simulink model "d_014"  (Simulink 5.1)
settings: Solver=ode45  StartTime=0.0  StopTime=10.0  RelTol=1e-3
libraries: fm_lib x30
settings Model: Creator=fmilano  LastModifiedBy=fmilano  ExtModeAutoUpdateStatusClock=off  SignalLoggingName=logsout  RTWOptions="-aEnforceIntegerDowncast=1 -aFoldNonRolledExpr=1 -aInlineInvariantSignals=1 -aInlineParameters=0 -aLocalBlockOutputs=1 -aRollThreshold=5 -aZeroInternalMemoryAtStartup=1 -aZeroExternalMemoryAtStartup=1 -aInitFltsAndDblsToZero=1 -aForceBlockIOInitOptimize=0 -aGenerateReport=0 -aGenCodeOnly=0 -aRTWVerbose=1 -aIncludeHyperlinkInReport=0 -aLaunchReport=0 -aGenerateTraceInfo=0  -aForceParamTrailComments=0 -aGenerateComments=1 -aIgnoreCustomStorageClasses=1 -aIncHierarchyInIds=0 -aMaxRTWIdLen=31 -aShowEliminatedStatements=0 -aIncDataTypeInIds=0 -aInsertBlockDesc=0 -aIgnoreTestpoints=0 -aSimulinkBlockComments=1 -aInlinedPrmAccess=\"Literals\"  -aSuppressErrorStatus=0 -aModelReferenceCompliant=1 -aParenthesesLevel=\"Nominal\" -aModelStepFunctionPrototypeControlCompliant=0 -aPortableWordSizes=0 -aParMdlRefBuildCompliant=0 -aSupportNonInlinedSFcns=1 -aSupportContinuousTime=1 -aSupportComplex=1 -aSupportNonFinite=1 -aSupportAbsoluteTime=1 -aMultiwordLength=2048 -aTargetPreCompLibLocation=\"\" -aTargetLibSuffix=\"\" -aTargetFunctionLibrary=\"ANSI_C\" -aTargetFcnLib=\"ansi_tfl_tmw.mat\" -aMultiInstanceERTCode=0 -aLogVarNameModifier=\"rt_\" -aERTFirstTimeCompliant=0 -aIsPILTarget=0 -aCombineOutputUpdateFcns=0 -aGenerateASAP2=0 -aGenerateClassInterface=0 -aGenerateTestInterfaces=0 -aGenerateSampleERTMain=0 -aGenerateFullHeader=1 -aUtilityFuncGeneration=\"Auto\" -aIncludeFileDelimiter=\"Auto\" -aIncludeMdlTerminateFcn=1 -aPurelyIntegerCode=0 -aAutosarCompliant=0 -aERTCustomFileBanners=0 -aRTWCAPIStates=0 -aRTWCAPIParams=0 -aRTWCAPISignals=0 -aMatFileLogging=1 -aCompOptLevelCompliant=0 -aCPPClassGenCompliant=0 -aExtModeIntrfLevel=\"Level1\" -aExtModeMexFile=\"ext_comm\" -aExtModeTransport=0 -aExtModeStaticAllocSize=1000000 -aExtModeTesting=0 -aExtModeStaticAlloc=0 -aExtMode=0 -aERTMultiwordLength=256 -aERTMultiwordTypeDef=\"System defined\"  -aGenerateTraceInfo=0 -aGenerateTraceInfo=0 -aGenerateTraceInfo=0 -aGenerateTraceInfo=0 -aPrefixModelToSubsysFcnNames=1 -aGenerateASAP2=0 -aRTWCAPIStates=0 -aRTWCAPIParams=0 -aRTWCAPISignals=0 -aExtModeMexFile=\"ext_comm\" -aExtModeTransport=0 -aExtModeStaticAllocSize=1000000 -aExtModeTesting=0 -aExtModeStaticAlloc=0 -aExtMode=0"

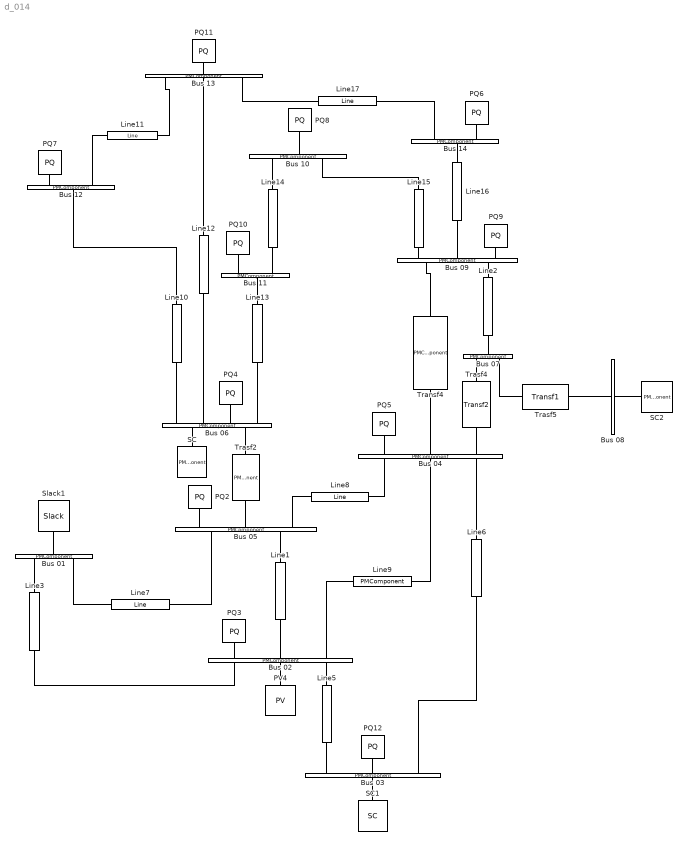
== system d_014 ==
  Bus 01 : PMComponent  Tag=PSATblock  Description=Connection  Orientation=down  PhysicalDomain=psatdomain  LeftPortType=p1  RightPortType=p1  LConnTagsString=__newl0  RConnTagsString=__newr0|__newr1  mask(Bus){in=1, out=2, p2q=69, p3_4q=[1.00  0.00], p5q=4, p6q=1}
      mask prompts: in "Number of inputs:"; out "Number of outputs:"; p2q "Voltage Rating [kV]"; p3_4q "Voltage initial guess [p.u.  rad]"; p5q "Area number"; p6q "Region number"
      mask help: Bus block.
      mask init:
      | fm_inout
      mask CallbackString: ||||fm_block|
      mask Display: plot([0 1 1 0 0],[0 0 1 1 0])
  Bus 02 : PMComponent  Tag=PSATblock  Description=Connection  Orientation=up  PhysicalDomain=psatdomain  LeftPortType=p1  RightPortType=p1  LConnTagsString=__newl0|__newl1|__newl2  RConnTagsString=__newr0|__newr1|__newr2  mask(Bus){in=3, out=3, p2q=69, p3_4q=[1.00  0.00], p5q=4, p6q=1}
      mask prompts: in "Number of inputs:"; out "Number of outputs:"; p2q "Voltage Rating [kV]"; p3_4q "Voltage initial guess [p.u.  rad]"; p5q "Area number"; p6q "Region number"
      mask help: Bus block.
      mask init:
      | fm_inout
      mask CallbackString: ||||fm_block|
      mask Display: plot([0 1 1 0 0],[0 0 1 1 0])
  Bus 03 : PMComponent  Tag=PSATblock  Description=Connection  Orientation=up  PhysicalDomain=psatdomain  LeftPortType=p1  RightPortType=p1  LConnTagsString=__newl0  RConnTagsString=__newr0|__newr1|__newr2  mask(Bus){in=1, out=3, p2q=69, p3_4q=[1.00  0.00], p5q=4, p6q=1}
      mask prompts: in "Number of inputs:"; out "Number of outputs:"; p2q "Voltage Rating [kV]"; p3_4q "Voltage initial guess [p.u.  rad]"; p5q "Area number"; p6q "Region number"
      mask help: Bus block.
      mask init:
      | fm_inout
      mask CallbackString: ||||fm_block|
      mask Display: plot([0 1 1 0 0],[0 0 1 1 0])
  Bus 04 : PMComponent  Tag=PSATblock  Description=Connection  Orientation=up  PhysicalDomain=psatdomain  LeftPortType=p1  RightPortType=p1  LConnTagsString=__newl0|__newl1|__newl2  RConnTagsString=__newr0|__newr1|__newr2  mask(Bus){in=3, out=3, p2q=69, p3_4q=[1.00  0.00], p5q=4, p6q=1}
      mask prompts: in "Number of inputs:"; out "Number of outputs:"; p2q "Voltage Rating [kV]"; p3_4q "Voltage initial guess [p.u.  rad]"; p5q "Area number"; p6q "Region number"
      mask help: Bus block.
      mask init:
      | fm_inout
      mask CallbackString: ||||fm_block|
      mask Display: plot([0 1 1 0 0],[0 0 1 1 0])
  Bus 05 : PMComponent  Tag=PSATblock  Description=Connection  Orientation=up  PhysicalDomain=psatdomain  LeftPortType=p1  RightPortType=p1  LConnTagsString=__newl0|__newl1  RConnTagsString=__newr0|__newr1|__newr2  mask(Bus){in=2, out=3, p2q=69, p3_4q=[1.00  0.00], p5q=4, p6q=1}
      mask prompts: in "Number of inputs:"; out "Number of outputs:"; p2q "Voltage Rating [kV]"; p3_4q "Voltage initial guess [p.u.  rad]"; p5q "Area number"; p6q "Region number"
      mask help: Bus block.
      mask init:
      | fm_inout
      mask CallbackString: ||||fm_block|
      mask Display: plot([0 1 1 0 0],[0 0 1 1 0])
  Bus 06 : PMComponent  Tag=PSATblock  Description=Connection  Orientation=up  PhysicalDomain=psatdomain  LeftPortType=p1  RightPortType=p1  LConnTagsString=__newl0|__newl1  RConnTagsString=__newr0|__newr1|__newr2|__newr3  mask(Bus){in=2, out=4, p2q=13.8, p3_4q=[1.00  0.00], p5q=2, p6q=1}
      mask prompts: in "Number of inputs:"; out "Number of outputs:"; p2q "Voltage Rating [kV]"; p3_4q "Voltage initial guess [p.u.  rad]"; p5q "Area number"; p6q "Region number"
      mask help: Bus block.
      mask init:
      | fm_inout
      mask CallbackString: ||||fm_block|
      mask Display: plot([0 1 1 0 0],[0 0 1 1 0])
  Bus 07 : PMComponent  Tag=PSATblock  Description=Connection  Orientation=up  PhysicalDomain=psatdomain  LeftPortType=p1  RightPortType=p1  LConnTagsString=__newl0|__newl1  RConnTagsString=__newr0  mask(Bus){in=2, out=1, p2q=13.8, p3_4q=[1.00  0.00], p5q=2, p6q=1}
      mask prompts: in "Number of inputs:"; out "Number of outputs:"; p2q "Voltage Rating [kV]"; p3_4q "Voltage initial guess [p.u.  rad]"; p5q "Area number"; p6q "Region number"
      mask help: Bus block.
      mask init:
      | fm_inout
      mask CallbackString: ||||fm_block|
      mask Display: plot([0 1 1 0 0],[0 0 1 1 0])
  Bus 08 : PMComponent  Tag=PSATblock  Description=Connection  Orientation=left  PhysicalDomain=psatdomain  LeftPortType=p1  RightPortType=p1  LConnTagsString=__newl0  RConnTagsString=__newr0  mask(Bus){in=1, out=1, p2q=18, p3_4q=[1.00  0.00], p5q=3, p6q=1}
      mask prompts: in "Number of inputs:"; out "Number of outputs:"; p2q "Voltage Rating [kV]"; p3_4q "Voltage initial guess [p.u.  rad]"; p5q "Area number"; p6q "Region number"
      mask help: Bus block.
      mask init:
      | fm_inout
      mask CallbackString: ||||fm_block|
      mask Display: plot([0 1 1 0 0],[0 0 1 1 0])
  Bus 09 : PMComponent  Tag=PSATblock  Description=Connection  Orientation=up  PhysicalDomain=psatdomain  LeftPortType=p1  RightPortType=p1  LConnTagsString=__newl0|__newl1  RConnTagsString=__newr0|__newr1|__newr2  mask(Bus){in=2, out=3, p2q=13.8, p3_4q=[1.00  0.00], p5q=2, p6q=1}
      mask prompts: in "Number of inputs:"; out "Number of outputs:"; p2q "Voltage Rating [kV]"; p3_4q "Voltage initial guess [p.u.  rad]"; p5q "Area number"; p6q "Region number"
      mask help: Bus block.
      mask init:
      | fm_inout
      mask CallbackString: ||||fm_block|
      mask Display: plot([0 1 1 0 0],[0 0 1 1 0])
  Bus 10 : PMComponent  Tag=PSATblock  Description=Connection  Orientation=up  PhysicalDomain=psatdomain  LeftPortType=p1  RightPortType=p1  LConnTagsString=__newl0|__newl1  RConnTagsString=__newr0  mask(Bus){in=2, out=1, p2q=13.8, p3_4q=[1.00  0.00], p5q=2, p6q=1}
      mask prompts: in "Number of inputs:"; out "Number of outputs:"; p2q "Voltage Rating [kV]"; p3_4q "Voltage initial guess [p.u.  rad]"; p5q "Area number"; p6q "Region number"
      mask help: Bus block.
      mask init:
      | fm_inout
      mask CallbackString: ||||fm_block|
      mask Display: plot([0 1 1 0 0],[0 0 1 1 0])
  Bus 11 : PMComponent  Tag=PSATblock  Description=Connection  Orientation=up  PhysicalDomain=psatdomain  LeftPortType=p1  RightPortType=p1  LConnTagsString=__newl0  RConnTagsString=__newr0|__newr1  mask(Bus){in=1, out=2, p2q=13.8, p3_4q=[1.00  0.00], p5q=2, p6q=1}
      mask prompts: in "Number of inputs:"; out "Number of outputs:"; p2q "Voltage Rating [kV]"; p3_4q "Voltage initial guess [p.u.  rad]"; p5q "Area number"; p6q "Region number"
      mask help: Bus block.
      mask init:
      | fm_inout
      mask CallbackString: ||||fm_block|
      mask Display: plot([0 1 1 0 0],[0 0 1 1 0])
  Bus 12 : PMComponent  Tag=PSATblock  Description=Connection  Orientation=up  PhysicalDomain=psatdomain  LeftPortType=p1  RightPortType=p1  LConnTagsString=__newl0  RConnTagsString=__newr0|__newr1  mask(Bus){in=1, out=2, p2q=13.8, p3_4q=[1.00  0.00], p5q=2, p6q=1}
      mask prompts: in "Number of inputs:"; out "Number of outputs:"; p2q "Voltage Rating [kV]"; p3_4q "Voltage initial guess [p.u.  rad]"; p5q "Area number"; p6q "Region number"
      mask help: Bus block.
      mask init:
      | fm_inout
      mask CallbackString: ||||fm_block|
      mask Display: plot([0 1 1 0 0],[0 0 1 1 0])
  Bus 13 : PMComponent  Tag=PSATblock  Description=Connection  Orientation=up  PhysicalDomain=psatdomain  LeftPortType=p1  RightPortType=p1  LConnTagsString=__newl0|__newl1|__newl2  RConnTagsString=__newr0  mask(Bus){in=3, out=1, p2q=13.8, p3_4q=[1.00  0.00], p5q=2, p6q=1}
      mask prompts: in "Number of inputs:"; out "Number of outputs:"; p2q "Voltage Rating [kV]"; p3_4q "Voltage initial guess [p.u.  rad]"; p5q "Area number"; p6q "Region number"
      mask help: Bus block.
      mask init:
      | fm_inout
      mask CallbackString: ||||fm_block|
      mask Display: plot([0 1 1 0 0],[0 0 1 1 0])
  Bus 14 : PMComponent  Tag=PSATblock  Description=Connection  Orientation=up  PhysicalDomain=psatdomain  LeftPortType=p1  RightPortType=p1  LConnTagsString=__newl0  RConnTagsString=__newr0|__newr1  mask(Bus){in=1, out=2, p2q=13.8, p3_4q=[1.00  0.00], p5q=2, p6q=1}
      mask prompts: in "Number of inputs:"; out "Number of outputs:"; p2q "Voltage Rating [kV]"; p3_4q "Voltage initial guess [p.u.  rad]"; p5q "Area number"; p6q "Region number"
      mask help: Bus block.
      mask init:
      | fm_inout
      mask CallbackString: ||||fm_block|
      mask Display: plot([0 1 1 0 0],[0 0 1 1 0])
  Line1 : fm_lib/Power Flow/Line  Tag=PSATblock  Description=Power Flow  Orientation=up  PhysicalDomain=psatdomain  SubClassName=unknown  LeftPortType=p1  RightPortType=p1  LConnTagsString=__newl0  RConnTagsString=__newr0  p3_4_5q="[100  69  60]"  p6q=0  p8q=0.05695  p9q=0.17388  p10q=0.034  p13_14_15q="[0.0  0.0  0.0]"  p16q=on
  Line10 : PMComponent  Tag=PSATblock  Description=Power Flow  Orientation=up  PhysicalDomain=psatdomain  LeftPortType=p1  RightPortType=p1  LConnTagsString=__newl0  RConnTagsString=__newr0  mask(Line){p3_4_5q=[100  13.8  60], p6q=0, p8q=0.12291, p9q=0.25581, p10q=0.00, p13_14_15q=[0.0  0.0  0.0], p16q=on}
      mask prompts: p3_4_5q "Power, Voltage and Frequency Ratings [MVA, kV, Hz]"; p6q "Length of line [km] (0 for p.u. parameters)"; p8q "Resistance [p.u. (Ohms/km)]"; p9q "Reactance [p.u. (H/km)]"; p10q "Susceptance [p.u. (F/km)]"; p13_14_15q "Imax, Pmax and Smax [p.u., p.u., p.u.]"; p16q "Connected"
      mask help: This block defines a pi model for a tree phase line.
      mask init:
      | [xp,yp] = fm_draw('pi');
      mask CallbackString: ||||||fm_block
      mask Display:
      | plot([-1  1  1 -1 -1],[-0.2 -0.2 0.2 0.2 -0.2])
      | color('blue')
      | plot(0.35*xp,0.2*yp)
  Line11 : fm_lib/Power Flow/Line  Tag=PSATblock  Description=Power Flow  PhysicalDomain=psatdomain  SubClassName=unknown  LeftPortType=p1  RightPortType=p1  LConnTagsString=__newl0  RConnTagsString=__newr0  p3_4_5q="[100  13.8  60]"  p6q=0  p8q=0.22092  p9q=0.19988  p10q=0.00  p13_14_15q="[0.0  0.0  0.0]"  p16q=on
  Line12 : fm_lib/Power Flow/Line  Tag=PSATblock  Description=Power Flow  Orientation=up  PhysicalDomain=psatdomain  SubClassName=unknown  LeftPortType=p1  RightPortType=p1  LConnTagsString=__newl0  RConnTagsString=__newr0  p3_4_5q="[100  13.8  60]"  p6q=0  p8q=0.06615  p9q=0.13027  p10q=0.00  p13_14_15q="[0.0  0.0  0.0]"  p16q=on
  Line13 : fm_lib/Power Flow/Line  Tag=PSATblock  Description=Power Flow  Orientation=up  PhysicalDomain=psatdomain  SubClassName=unknown  LeftPortType=p1  RightPortType=p1  LConnTagsString=__newl0  RConnTagsString=__newr0  p3_4_5q="[100  13.8  60]"  p6q=0  p8q=0.09498  p9q=0.1989  p10q=0.00  p13_14_15q="[0.0  0.0  0.0]"  p16q=on
  Line14 : fm_lib/Power Flow/Line  Tag=PSATblock  Description=Power Flow  Orientation=up  PhysicalDomain=psatdomain  SubClassName=unknown  LeftPortType=p1  RightPortType=p1  LConnTagsString=__newl0  RConnTagsString=__newr0  p3_4_5q="[100  13.8  60]"  p6q=0  p8q=0.08205  p9q=0.19207  p10q=0.00  p13_14_15q="[0.0  0.0  0.0]"  p16q=on
  Line15 : fm_lib/Power Flow/Line  Tag=PSATblock  Description=Power Flow  Orientation=up  PhysicalDomain=psatdomain  SubClassName=unknown  LeftPortType=p1  RightPortType=p1  LConnTagsString=__newl0  RConnTagsString=__newr0  p3_4_5q="[100  13.8  60]"  p6q=0  p8q=0.03181  p9q=0.0845  p10q=0.00  p13_14_15q="[0.0  0.0  0.0]"  p16q=on
  Line16 : fm_lib/Power Flow/Line  Tag=PSATblock  Description=Power Flow  Orientation=up  PhysicalDomain=psatdomain  SubClassName=unknown  LeftPortType=p1  RightPortType=p1  LConnTagsString=__newl0  RConnTagsString=__newr0  p3_4_5q="[100  13.8  60]"  p6q=0  p8q=0.12711  p9q=0.27038  p10q=0.00  p13_14_15q="[0.0  0.0  0.0]"  p16q=on
  Line17 : fm_lib/Power Flow/Line  Tag=PSATblock  Description=Power Flow  Orientation=left  PhysicalDomain=psatdomain  SubClassName=unknown  LeftPortType=p1  RightPortType=p1  LConnTagsString=__newl0  RConnTagsString=__newr0  p3_4_5q="[100  13.8  60]"  p6q=0  p8q=0.17093  p9q=0.34802  p10q=0.00  p13_14_15q="[0.0  0.0  0.0]"  p16q=on
  Line2 : fm_lib/Power Flow/Line  Tag=PSATblock  Description=Power Flow  Orientation=up  PhysicalDomain=psatdomain  SubClassName=unknown  LeftPortType=p1  RightPortType=p1  LConnTagsString=__newl0  RConnTagsString=__newr0  p3_4_5q="[100  13.8  60]"  p6q=0  p8q=0.00  p9q=0.11001  p10q=0.00  p13_14_15q="[0.0  0.0  0.0]"  p16q=on
  Line3 : fm_lib/Power Flow/Line  Tag=PSATblock  Description=Power Flow  Orientation=down  PhysicalDomain=psatdomain  SubClassName=unknown  LeftPortType=p1  RightPortType=p1  LConnTagsString=__newl0  RConnTagsString=__newr0  p3_4_5q="[100  69  60]"  p6q=0  p8q=0.01938  p9q=0.05917  p10q=0.0528  p13_14_15q="[0.0  0.0  0.0]"  p16q=on
  Line5 : fm_lib/Power Flow/Line  Tag=PSATblock  Description=Power Flow  Orientation=up  PhysicalDomain=psatdomain  SubClassName=unknown  LeftPortType=p1  RightPortType=p1  LConnTagsString=__newl0  RConnTagsString=__newr0  p3_4_5q="[100  69  60]"  p6q=0  p8q=0.04699  p9q=0.19797  p10q=0.0438  p13_14_15q="[0.0  0.0  0.0]"  p16q=on
  Line6 : fm_lib/Power Flow/Line  Tag=PSATblock  Description=Power Flow  Orientation=up  PhysicalDomain=psatdomain  SubClassName=unknown  LeftPortType=p1  RightPortType=p1  LConnTagsString=__newl0  RConnTagsString=__newr0  p3_4_5q="[100  69  60]"  p6q=0  p8q=0.06701  p9q=0.17103  p10q=0.0346  p13_14_15q="[0.0  0.0  0.0]"  p16q=on
  Line7 : fm_lib/Power Flow/Line  Tag=PSATblock  Description=Power Flow  PhysicalDomain=psatdomain  SubClassName=unknown  LeftPortType=p1  RightPortType=p1  LConnTagsString=__newl0  RConnTagsString=__newr0  p3_4_5q="[100  69  60]"  p6q=0  p8q=0.05403  p9q=0.22304  p10q=0.0492  p13_14_15q="[0.0  0.0  0.0]"  p16q=on
  Line8 : fm_lib/Power Flow/Line  Tag=PSATblock  Description=Power Flow  PhysicalDomain=psatdomain  SubClassName=unknown  LeftPortType=p1  RightPortType=p1  LConnTagsString=__newl0  RConnTagsString=__newr0  p3_4_5q="[100  69  60]"  p6q=0  p8q=0.01335  p9q=0.04211  p10q=0.0128  p13_14_15q="[0.0  0.0  0.0]"  p16q=on
  Line9 : PMComponent  Tag=PSATblock  Description=Power Flow  PhysicalDomain=psatdomain  LeftPortType=p1  RightPortType=p1  LConnTagsString=__newl0  RConnTagsString=__newr0  mask(Line){p3_4_5q=[100  69  60], p6q=0, p8q=0.05811, p9q=0.17632, p10q=0.0374, p13_14_15q=[0.0  0.0  0.0], p16q=on}
      mask prompts: p3_4_5q "Power, Voltage and Frequency Ratings [MVA, kV, Hz]"; p6q "Length of line [km] (0 for p.u. parameters)"; p8q "Resistance [p.u. (Ohms/km)]"; p9q "Reactance [p.u. (H/km)]"; p10q "Susceptance [p.u. (F/km)]"; p13_14_15q "Imax, Pmax and Smax [p.u., p.u., p.u.]"; p16q "Connected"
      mask help: This block defines a pi model for a tree phase line.
      mask init:
      | [xp,yp] = fm_draw('pi');
      mask CallbackString: ||||||fm_block
      mask Display:
      | plot([-1  1  1 -1 -1],[-0.2 -0.2 0.2 0.2 -0.2])
      | color('blue')
      | plot(0.35*xp,0.2*yp)
  PQ10 : fm_lib/Power Flow/PQ  Tag=PSATblock  Description=Power Flow  Orientation=up  PhysicalDomain=psatdomain  SubClassName=unknown  LeftPortType=p1  RightPortType=p1  LConnTagsString=__newl0  p2_3q="[100  13.8]"  p4_5q="[1.4*0.035  1.4*0.018]"  p6_7q="[1.2  0.8]"  p8q=off  p9q=on
  PQ11 : fm_lib/Power Flow/PQ  Tag=PSATblock  Description=Power Flow  Orientation=up  PhysicalDomain=psatdomain  SubClassName=unknown  LeftPortType=p1  RightPortType=p1  LConnTagsString=__newl0  p2_3q="[100  13.8]"  p4_5q="[1.4*0.135  1.4*0.058]"  p6_7q="[1.2  0.8]"  p8q=off  p9q=on
  PQ12 : fm_lib/Power Flow/PQ  Tag=PSATblock  Description=Power Flow  Orientation=up  PhysicalDomain=psatdomain  SubClassName=unknown  LeftPortType=p1  RightPortType=p1  LConnTagsString=__newl0  p2_3q="[100  69]"  p4_5q="[1.4*0.942  1.4*0.19]"  p6_7q="[1.2  0.8]"  p8q=off  p9q=on
  PQ2 : fm_lib/Power Flow/PQ  Tag=PSATblock  Description=Power Flow  Orientation=up  PhysicalDomain=psatdomain  SubClassName=unknown  LeftPortType=p1  RightPortType=p1  LConnTagsString=__newl0  p2_3q="[100  69]"  p4_5q="[1.4*0.076  1.4*0.016]"  p6_7q="[1.2  0.8]"  p8q=off  p9q=on
  PQ3 : fm_lib/Power Flow/PQ  Tag=PSATblock  Description=Power Flow  Orientation=up  PhysicalDomain=psatdomain  SubClassName=unknown  LeftPortType=p1  RightPortType=p1  LConnTagsString=__newl0  p2_3q="[100  69]"  p4_5q="[1.4*0.217  1.4*0.127]"  p6_7q="[1.2  0.8]"  p8q=off  p9q=on
  PQ4 : fm_lib/Power Flow/PQ  Tag=PSATblock  Description=Power Flow  Orientation=up  PhysicalDomain=psatdomain  SubClassName=unknown  LeftPortType=p1  RightPortType=p1  LConnTagsString=__newl0  p2_3q="[100  13.8]"  p4_5q="[1.4*0.112  1.4*0.075]"  p6_7q="[1.2  0.8]"  p8q=off  p9q=on
  PQ5 : fm_lib/Power Flow/PQ  Tag=PSATblock  Description=Power Flow  Orientation=up  PhysicalDomain=psatdomain  SubClassName=unknown  LeftPortType=p1  RightPortType=p1  LConnTagsString=__newl0  p2_3q="[100  69]"  p4_5q="[1.4*0.478  1.4*0.04]"  p6_7q="[1.2  0.8]"  p8q=off  p9q=on
  PQ6 : fm_lib/Power Flow/PQ  Tag=PSATblock  Description=Power Flow  Orientation=up  PhysicalDomain=psatdomain  SubClassName=unknown  LeftPortType=p1  RightPortType=p1  LConnTagsString=__newl0  p2_3q="[100  13.8]"  p4_5q="[1.4*0.149  1.4*0.05]"  p6_7q="[1.2  0.8]"  p8q=off  p9q=on
  PQ7 : fm_lib/Power Flow/PQ  Tag=PSATblock  Description=Power Flow  Orientation=up  PhysicalDomain=psatdomain  SubClassName=unknown  LeftPortType=p1  RightPortType=p1  LConnTagsString=__newl0  p2_3q="[100  13.8]"  p4_5q="[1.4*0.061  1.4*0.016]"  p6_7q="[1.2  0.8]"  p8q=off  p9q=on
  PQ8 : fm_lib/Power Flow/PQ  Tag=PSATblock  Description=Power Flow  Orientation=up  PhysicalDomain=psatdomain  SubClassName=unknown  LeftPortType=p1  RightPortType=p1  LConnTagsString=__newl0  p2_3q="[100  13.8]"  p4_5q="[1.4*0.09  1.4*0.058]"  p6_7q="[1.2  0.8]"  p8q=off  p9q=on
  PQ9 : fm_lib/Power Flow/PQ  Tag=PSATblock  Description=Power Flow  Orientation=up  PhysicalDomain=psatdomain  SubClassName=unknown  LeftPortType=p1  RightPortType=p1  LConnTagsString=__newl0  p2_3q="[100  13.8]"  p4_5q="[1.4*0.295  1.4*0.166]"  p6_7q="[1.2  0.8]"  p8q=off  p9q=on
  PV4 : fm_lib/Power Flow/PV  Tag=PSATblock  Description=Power Flow  Orientation=up  PhysicalDomain=psatdomain  SubClassName=unknown  LeftPortType=p1  RightPortType=p1  RConnTagsString=__newr0  p2_3q="[100  69]"  p4q=0.4  p5q=1.045  p6_7q="[0.5  -0.4]"  p8_9q="[1.2  0.8]"  p10q=1  p11q=on
  SC : PMComponent  Tag=PSATblock  Description=Power Flow  Orientation=up  PhysicalDomain=psatdomain  LeftPortType=p1  RightPortType=p1  RConnTagsString=__newr0  mask(PV){p2_3q=[100  13.8], p5q=1.07, p6_7q=[0.24  -0.06], p8_9q=[1.2  0.8], p10q=1, p11q=on}
      mask prompts: p2_3q "Power and Voltage Ratings [MVA, kV]"; p5q "Voltage Magnitude [p.u.]"; p6_7q "Qmax & Qmin [p.u.  p.u.]"; p8_9q "Vmax & Vmin [p.u.  p.u.]"; p10q "Loss Participation Coefficient"; p11q "Connected"
      mask help:
      | This block defines a static synchronous compensator:
      | P = 0
      | V = Vdes
      mask init:
      | [x,y] = fm_draw('circle');
      | [xc,yc] = fm_draw('C');
      mask CallbackString: |||||fm_block
      mask Display:
      | plot(x,y,[-0.25 -0.25],[-0.25 0.25])
      | color('blue')
      | plot(0.5*xc-0.25,yc)
  SC1 : fm_lib/Power Flow/SC  Tag=PSATblock  Description=Power Flow  Orientation=up  PhysicalDomain=psatdomain  SubClassName=unknown  LeftPortType=p1  RightPortType=p1  RConnTagsString=__newr0  p2_3q="[100  69]"  p5q=1.01  p6_7q="[0.4  0.0]"  p8_9q="[1.2  0.8]"  p10q=1  p11q=on
  SC2 : PMComponent  Tag=PSATblock  Description=Power Flow  Orientation=left  PhysicalDomain=psatdomain  LeftPortType=p1  RightPortType=p1  RConnTagsString=__newr0  mask(PV){p2_3q=[100  18], p5q=1.09, p6_7q=[0.24  -0.06], p8_9q=[1.2  0.8], p10q=1, p11q=on}
      mask prompts: p2_3q "Power and Voltage Ratings [MVA, kV]"; p5q "Voltage Magnitude [p.u.]"; p6_7q "Qmax & Qmin [p.u.  p.u.]"; p8_9q "Vmax & Vmin [p.u.  p.u.]"; p10q "Loss Participation Coefficient"; p11q "Connected"
      mask help:
      | This block defines a static synchronous compensator:
      | P = 0
      | V = Vdes
      mask init:
      | [x,y] = fm_draw('circle');
      | [xc,yc] = fm_draw('C');
      mask CallbackString: |||||fm_block
      mask Display:
      | plot(x,y,[-0.25 -0.25],[-0.25 0.25])
      | color('blue')
      | plot(0.5*xc-0.25,yc)
  Slack1 : fm_lib/Power Flow/Slack  Tag=PSATblock  Description=Power Flow  Orientation=down  PhysicalDomain=psatdomain  SubClassName=unknown  LeftPortType=p1  RightPortType=p1  RConnTagsString=__newr0  p2_3q="[100  69]"  p4q=1.06  p5q=0.00  p6_7q="[9.9  -9.9]"  p8_9q="[1.2  0.8]"  p10q=2.324  p11q=1  p12q=on  p13q=on
  Transf4 : PMComponent  Tag=PSATblock  Description=Power Flow  Orientation=up  PhysicalDomain=psatdomain  LeftPortType=p1  RightPortType=p1  LConnTagsString=__newl0  RConnTagsString=__newr0  mask(Line){p3_4_5q=[100  69  60], p7q=69/13.8, p8q=0.005, p9q=0.55618, p11q=0.969, p12q=5.00, p13_14_15q=[0.0  0.0  0.0], p16q=on}
      mask prompts: p3_4_5q "Power, Voltage and Frequency Ratings [MVA, kV, Hz]"; p7q "Primary and secondary voltage ratio [kV/kV]"; p8q "Resistance [p.u.]"; p9q "Reactance [p.u.]"; p11q "Fixed tap ratio [p.u./p.u.]"; p12q "Fixed phase shift [deg]"; p13_14_15q "Imax, Pmax and Smax [p.u. p.u. p.u.]"; p16q "Connected"
      mask help: This block defines a transformer with constant phase shifter and constant tap ratio.
      mask init:
      | [x,y] = fm_draw('circle');
      | [xa,ya] = fm_draw('a');
      | [x2,y2] = fm_draw('2');
      mask CallbackString: |||||||fm_block
      mask Display:
      | plot(x,y,x+1.4,y,[-1 -1.3],[0 0],[2.4 2.7],[0 0],[2.7 2.7 4 4 2.7],[-0.5 0.5 0.5 -0.5 -0.5],[4 4.3],[0 0])
      | color('green')
      | plot([-0.8 0.7],[-1.2 1.2],[0.5 0.7],[1.1 1.2],[0.7 0.7],[1.0 1.2])
      | plot(1.5+0.65*x2,0.65*y2)
      | color('red')
      | plot(3.35+0.2*xa,-0.1+0.15*ya)
  Trasf2 : PMComponent  Tag=PSATblock  Description=Power Flow  Orientation=up  PhysicalDomain=psatdomain  LeftPortType=p1  RightPortType=p1  LConnTagsString=__newl0  RConnTagsString=__newr0  mask(Line){p3_4_5q=[100  69  60], p7q=69/13.8, p8q=0.00, p9q=0.25202, p11q=0.932, p13_14_15q=[0.0  0.0  0.0], p16q=on}
      mask prompts: p3_4_5q "Power, Voltage and Frequency Ratings [MVA, kV, Hz]"; p7q "Primary and secondary voltage ratio [kV/kV]"; p8q "Resistance [p.u.]"; p9q "Reactance [p.u.]"; p11q "Fixed tap ratio [p.u./p.u.]"; p13_14_15q "Imax, Pmax and Smax  [p.u., p.u., p.u.]"; p16q "Connected"
      mask help: This block defines a transformer with constant tap ratio.
      mask init:
      | [x,y] = fm_draw('circle');
      | [x2,y2] = fm_draw('2');
      mask CallbackString: ||||||fm_block
      mask Display:
      | plot(x,y,x+1.4,y,[-1 -1.3],[0 0],[2.4 2.7],[0 0])
      | color('green')
      | plot([-0.8 0.7],[-1.2 1.2],[0.5 0.7],[1.1 1.2],[0.7 0.7],[1.0 1.2])
      | plot(1.5+0.65*x2,0.65*y2)
  Trasf4 : fm_lib/Power Flow/Transf2  Tag=PSATblock  Description=Power Flow  Orientation=up  PhysicalDomain=psatdomain  SubClassName=unknown  LeftPortType=p1  RightPortType=p1  LConnTagsString=__newl0  RConnTagsString=__newr0  p3_4_5q="[100  69  60]"  p7q=69/13.8  p8q=0.0  p9q=0.20912  p11q=0.978  p13_14_15q="[0.0  0.0  0.0]"  p16q=on
  Trasf5 : fm_lib/Power Flow/Transf1  Tag=PSATblock  Description=Power Flow  Orientation=left  PhysicalDomain=psatdomain  SubClassName=unknown  LeftPortType=p1  RightPortType=p1  LConnTagsString=__newl0  RConnTagsString=__newr0  p3_4_5q="[100  18  60]"  p7q=18/13.8  p8q=0.00  p9q=0.17615  p13_14_15q="[0.0  0.0  0.0]"  p16q=on
  connections:
  Trasf2/RConn1 -- Bus 06/LConn2
  Line5/RConn1 -- Bus 02/LConn3
  Line14/RConn1 -- Bus 10/LConn1
  Bus 11/RConn2 -- Line14/LConn1
  Bus 14/RConn1 -- Line17/LConn1
  Line17/RConn1 -- Bus 13/LConn3
  Line16/RConn1 -- Bus 14/LConn1
  Bus 09/RConn2 -- Line16/LConn1
  Bus 14/RConn2 -- PQ6/LConn1
  Bus 09/RConn1 -- Line15/LConn1
  Line15/RConn1 -- Bus 10/LConn2
  Bus 11/RConn1 -- PQ10/LConn1
  Line13/RConn1 -- Bus 11/LConn1
  Bus 06/RConn4 -- Line13/LConn1
  Line12/RConn1 -- Bus 13/LConn2
  Bus 06/RConn2 -- Line12/LConn1
  Line10/RConn1 -- Bus 12/LConn1
  Bus 06/RConn1 -- Line10/LConn1
  Line11/RConn1 -- Bus 13/LConn1
  Bus 12/RConn2 -- Line11/LConn1
  Bus 12/RConn1 -- PQ7/LConn1
  Bus 13/RConn1 -- PQ11/LConn1
  Transf4/RConn1 -- Bus 09/LConn1
  Bus 09/RConn3 -- PQ9/LConn1
  SC2/RConn1 -- Bus 08/LConn1
  SC1/RConn1 -- Bus 03/LConn1
  Slack1/RConn1 -- Bus 01/LConn1
  Bus 08/RConn1 -- Trasf5/LConn1
  Trasf5/RConn1 -- Bus 07/LConn2
  Line2/RConn1 -- Bus 09/LConn2
  Bus 07/RConn1 -- Line2/LConn1
  Trasf4/RConn1 -- Bus 07/LConn1
  Bus 04/RConn3 -- Trasf4/LConn1
  Bus 02/RConn3 -- Line9/LConn1
  Line9/RConn1 -- Bus 04/LConn2
  Line8/RConn1 -- Bus 04/LConn1
  Bus 05/RConn3 -- Line8/LConn1
  Bus 06/RConn3 -- PQ4/LConn1
  Bus 05/RConn1 -- PQ2/LConn1
  Bus 01/RConn2 -- Line7/LConn1
  Line7/RConn1 -- Bus 05/LConn1
  Bus 04/RConn1 -- PQ5/LConn1
  Bus 04/RConn2 -- Transf4/LConn1
  Line6/RConn1 -- Bus 04/LConn3
  Bus 03/RConn3 -- Line6/LConn1
  Bus 03/RConn2 -- PQ12/LConn1
  Bus 03/RConn1 -- Line5/LConn1
  Bus 05/RConn2 -- Trasf2/LConn1
  Line1/RConn1 -- Bus 05/LConn2
  Line3/RConn1 -- Bus 02/LConn1
  Bus 01/RConn1 -- Line3/LConn1
  Bus 02/RConn2 -- Line1/LConn1
  Bus 02/RConn1 -- PQ3/LConn1
  Bus 10/RConn1 -- PQ8/LConn1
  PV4/RConn1 -- Bus 02/LConn2
  SC/RConn1 -- Bus 06/LConn1
